simulink model "Current_Controller_Design"  (R2024b)
settings: Solver=VariableStepAuto  StartTime=0.0  StopTime=0.1  RelTol=1e-3
values from neighbouring files (symbols this model uses):
  B = 0    [DC_Motor_Project.m]
  J = 0.00252    [DC_Motor_Project.m]
  K_ic = Ra * W_cc    (= 260)    [DC_Motor_Project.m]
  K_pc = La * W_cc    (= 1.7)    [DC_Motor_Project.m]
  Kac = 1 / K_pc    (= 0.588235294118)    [DC_Motor_Project.m]
  Kt = Te_rated / Ia_rated    (= 0.424752712124)    [DC_Motor_Project.m]
  La = 1.7e-3    (= 0.0017)    [DC_Motor_Project.m]
  Ra = 0.26    [DC_Motor_Project.m]
settings Model: Creator=LEGION  LastModifiedBy=LEGION

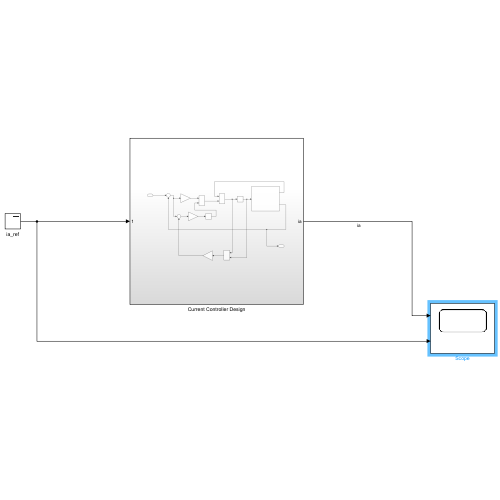
[thumbnail: Simulink's stored preview of the top-level diagram]
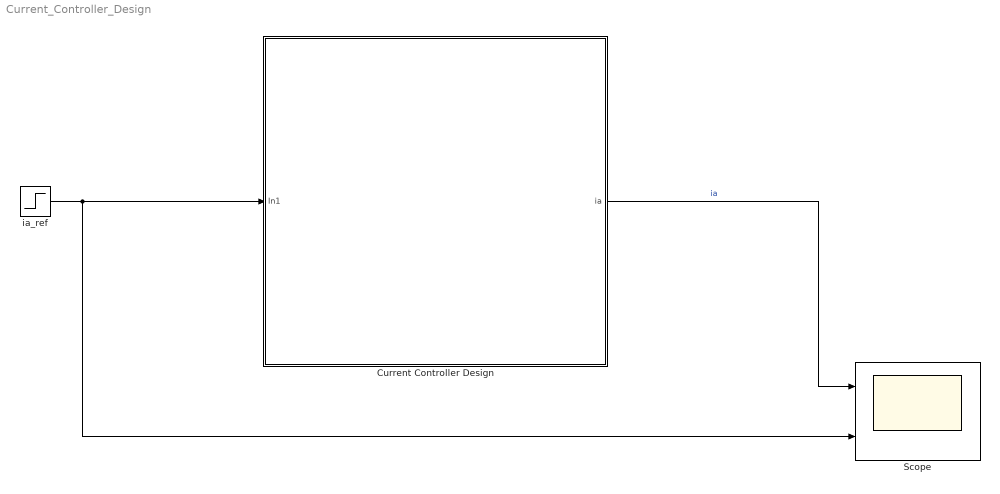
== system Current_Controller_Design ==
  Current Controller Design : Subsystem
  Scope : Scope  NumInputPorts=2
  ia_ref : Step  Time=0.01  After=10  SampleTime=0
  wires:
  ia_ref/1 -> Scope/2, Current Controller Design/1(In1)
  Current Controller Design/1(ia) -> Scope/1  "ia"

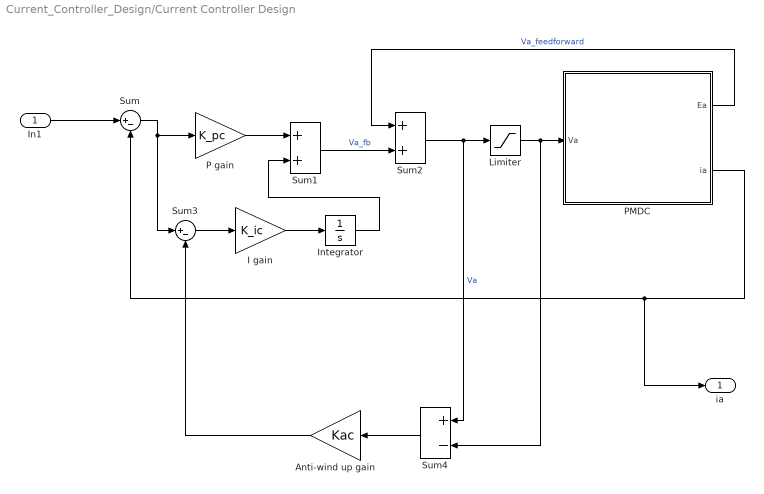
== system Current_Controller_Design/Current Controller Design ==
  In1 : Inport
  Anti-wind up gain : Gain  Gain=Kac
  I gain : Gain  Gain=K_ic
  Integrator : Integrator
  Limiter : Saturate  UpperLimit=220  LowerLimit=-220
  P gain : Gain  Gain=K_pc
  PMDC : Subsystem
  Sum : Sum  Inputs=|+-
  Sum1 : Sum
  Sum2 : Sum
  Sum3 : Sum  Inputs=|+-
  Sum4 : Sum  Inputs=+-
  ia : Outport
  wires:
  PMDC/2(ia) -> ia/1, Sum/2
  Integrator/1 -> Sum1/2
  Sum/1 -> Sum3/1, P gain/1
  I gain/1 -> Integrator/1
  Anti-wind up gain/1 -> Sum3/2
  P gain/1 -> Sum1/1
  Limiter/1 -> Sum4/2, PMDC/1(Va)
  In1/1 -> Sum/1
  Sum4/1 -> Anti-wind up gain/1
  PMDC/1(Ea) -> Sum2/1  "Va_feedforward"
  Sum1/1 -> Sum2/2  "Va_fb"
  Sum3/1 -> I gain/1
  Sum2/1 -> Sum4/1, Limiter/1  "Va"

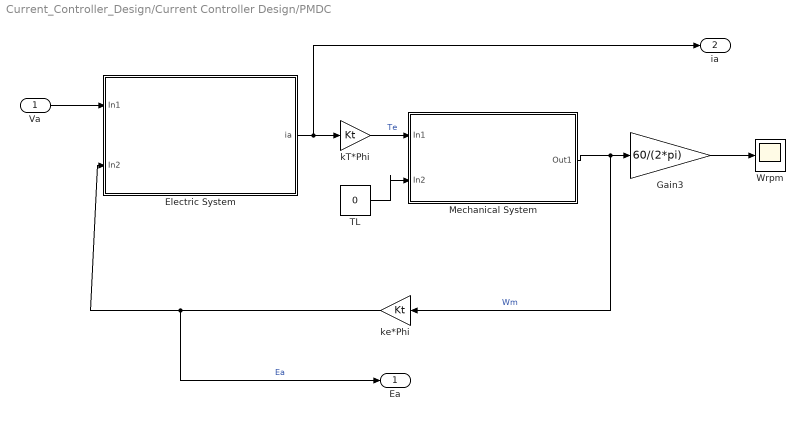
== system Current_Controller_Design/Current Controller Design/PMDC ==
  Va : Inport
  Electric System : Subsystem
  Gain3 : Gain  Gain=60/(2*pi)
  Mechanical System : Subsystem
  TL : Constant  Value=0
  Wrpm : Scope
  kT*Phi : Gain  Gain=Kt
  ke*Phi : Gain  Gain=Kt
  Ea : Outport
  ia : Outport  Port=2
  wires:
  ke*Phi/1 -> Ea/1, Electric System/2(In2)  "Ea"
  kT*Phi/1 -> Mechanical System/1(In1)  "Te"
  Mechanical System/1(Out1) -> ke*Phi/1, Gain3/1  "Wm"
  Gain3/1 -> Wrpm/1
  Electric System/1(ia) -> ia/1, kT*Phi/1
  TL/1 -> Mechanical System/2(In2)
  Va/1 -> Electric System/1(In1)

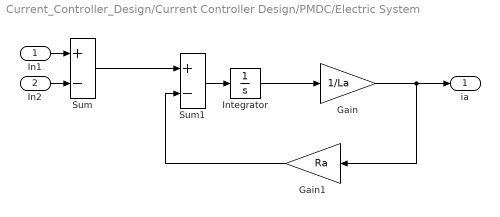
== system Current_Controller_Design/Current Controller Design/PMDC/Electric System ==
  In1 : Inport
  In2 : Inport  Port=2
  Gain : Gain  Gain=1/La
  Gain1 : Gain  Gain=Ra
  Integrator : Integrator
  Sum : Sum  Inputs=+-
  Sum1 : Sum  Inputs=+-
  ia : Outport
  wires:
  Sum1/1 -> Integrator/1
  In1/1 -> Sum/1
  Gain1/1 -> Sum1/2
  Gain/1 -> ia/1, Gain1/1
  Sum/1 -> Sum1/1
  Integrator/1 -> Gain/1
  In2/1 -> Sum/2

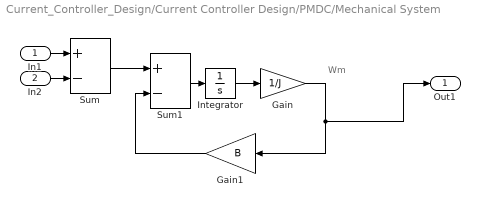
== system Current_Controller_Design/Current Controller Design/PMDC/Mechanical System ==
  note: Wm
  In1 : Inport
  In2 : Inport  Port=2
  Gain : Gain  Gain=1/J
  Gain1 : Gain  Gain=B
  Integrator : Integrator
  Sum : Sum  Inputs=+-
  Sum1 : Sum  Inputs=+-
  Out1 : Outport
  wires:
  Gain/1 -> Out1/1, Gain1/1
  Sum1/1 -> Integrator/1
  Sum/1 -> Sum1/1
  In1/1 -> Sum/1
  Gain1/1 -> Sum1/2
  Integrator/1 -> Gain/1
  In2/1 -> Sum/2
